simulink model "MOD_Hbridge_Ctrl"  (R2018b)
settings: Solver=VariableStepDiscrete  StartTime=0  StopTime=30  RelTol=1e-3
PreLoadFcn:
  | if(exist('MBDS_ModelCallback', 'file'))
  |    MBDS_ModelCallback('PreLoad');
  | end
PostLoadFcn:
  | if(exist('MBDS_ModelCallback', 'file'))
  |    MBDS_ModelCallback('PostLoad');
  | end
InitFcn:
  | if(exist('MBDS_ModelCallback', 'file'))
  |    MBDS_ModelCallback('Init');
  | end
StartFcn:
  | if(exist('MBDS_ModelCallback', 'file'))
  |    MBDS_ModelCallback('Start');
  | end
StopFcn:
  | if(exist('MBDS_ModelCallback', 'file'))
  |    MBDS_ModelCallback('Stop');
  | end
undefined symbols (not defined in the file): sigbuilder_block
libraries: simulink x1
(part 1 of 2)
PreSaveFcn:
  | if(exist('MBDS_ModelCallback', 'file'))
  |    MBDS_ModelCallback('PreSave');
  | end
CloseFcn:
  | if(exist('MBDS_ModelCallback', 'file'))
  |    MBDS_ModelCallback('Close');
  | end
Description:
  | Design model of an MBDS Module
settings Model: IsTargetCode=false  MBDS_Version=08.20  Creator=Denis Cerchiaro (uidu1522)  LastModifiedBy=uidu1522
settings ConfigSet: Description=MBDS configuration set optimized for simulation of model designs for automotive embedded systems.
settings SolverCC: MinimalZcImpactIntegration=on
settings DataIOCC: MaxDataPoints=100  SaveFormat=StructureWithTime  SaveOutput=off  DSMLogging=off  VisualizeSimOutput=off  SaveTime=off  SignalLoggingName=LogSignals
settings OptimizationCC: UseDivisionForNetSlopeComputation=UseDivisionForReciprocalsOfIntegersOnly  UseFloatMulNetSlope=on  DefaultUnderspecifiedDataType=single  OptimizeBlockIOStorage=off  BufferReuse=off  GlobalBufferReuse=off  StrengthReduction=on  ExpressionFolding=off  ExpressionDepthLimit=2147483647  LocalBlockOutputs=off  EfficientFloat2IntCast=on  LifeSpan=inf  BufferReusableBoundary=off  OptimizeBlockOrder=speed  OptimizeDataStoreBuffers=off  BusAssignmentInplaceUpdate=off  LabelGuidedReuse=on
settings DebuggingCC: SignalInfNanChecking=error  AlgebraicLoopMsg=error  ArtificialAlgebraicLoopMsg=error  UnderspecifiedInitializationDetection=Classic  CheckExecutionContextPreStartOutputMsg=on  CheckExecutionContextRuntimeOutputMsg=on  BlockPriorityViolationMsg=error  MinStepSizeMsg=error  TimeAdjustmentMsg=warning  SolverPrmCheckMsg=error  InheritedTsInSrcMsg=none  SingleTaskRateTransMsg=error  TasksWithSamePriorityMsg=error  SigSpecEnsureSampleTimeMsg=error  CheckMatrixSingularityMsg=error  ParameterUnderflowMsg=error  ParameterTunabilityLossMsg=error  FixptConstUnderflowMsg=warning  FixptConstOverflowMsg=warning  FixptConstPrecisionLossMsg=warning  VectorMatrixConversionMsg=error  SignalLabelMismatchMsg=warning  SFcnCompatibilityMsg=error  FrameProcessingCompatibilityMsg=warning  UniqueDataStoreMsg=error  BusObjectLabelMismatch=error  RootOutportRequireBusObject=error  AllowSymbolicDim=off  ModelReferenceIOMsg=error  ModelReferenceIOMismatchMessage=error  UnknownTsInhSupMsg=error  ModelReferenceDataLoggingMessage=error  StateNameClashWarn=warning  SimStateOlderReleaseMsg=warning  StrictBusMsg=ErrorOnBusTreatedAsVector  NonBusSignalsTreatedAsBus=error  SFInvalidInputDataAccessInChartInitDiag=error  SFTransitionOutsideNaturalParentDiag=error  SFUnreachableExecutionPathDiag=error  SFUndirectedBroadcastEventsDiag=error  SFTransitionActionBeforeConditionDiag=error  SFTemporalDelaySmallerThanSampleTimeDiag=error  SFExecutionAtInitializationDiag=none
settings HardwareCC: ProdBitPerPointer=32  ProdBitPerSizeT=32  ProdBitPerPtrDiffT=32  ProdLargestAtomicInteger=Long  ProdEndianess=BigEndian  ProdWordSize=32  ProdLongLongMode=on  ProdHWDeviceType=Custom Processor  TargetHWDeviceType=32-bit Generic
settings ModelReferenceCC: PropagateSignalLabelsOutOfModel=off
settings SFSimCC: SimUseLocalCustomCode=off  SimGenImportedTypeDefs=on  CompileTimeRecursionLimit=0  EnableRuntimeRecursion=off  MATLABDynamicMemAlloc=off  DefaultCustomCodeFunctionArrayLayout=Column-major
settings RTWCC: SystemTargetFile=MBDS.tlc  GenCodeOnly=on  TemplateMakefile=MBDS.tmf  Description=MBDS Target  GenerateReport=on  RTWUseLocalCustomCode=off  IncludeHyperlinkInReport=on  LaunchReport=on  GenerateTraceReport=on  GenerateTraceReportSl=on  GenerateTraceReportSf=on  GenerateTraceReportEml=on  GenerateCodeMetricsReport=on  RTWCompilerOptimization=on
settings CodeAppCC: ForceParamTrailComments=on  IgnoreCustomStorageClasses=off  OperatorAnnotations=on  SimulinkDataObjDesc=on  SFDataObjDesc=on  MangleLength=2  CustomSymbolStrType=$N$R$M  CustomSymbolStrFcn=$R$M  CustomSymbolStrUtil=$n$C  InsertBlockDesc=on  StateflowObjectComments=on  MATLABSourceComments=on  ReqsInCode=on  UseSimReservedNames=on
settings STFCustomTargetCC: UtilityFuncGeneration=Shared location  MultiwordLength=256  DynamicStringBufferSize=2  InferredTypesCompatibility=on  ModelReferenceCompliant=off  IncludeMdlTerminateFcn=off  CombineOutputUpdateFcns=on  CombineSignalStateStructs=on  SuppressErrorStatus=on  ERTCustomFileBanners=on  SupportComplex=off  SupportContinuousTime=off  SupportNonInlinedSFcns=off  RemoveDisableFunc=on  RemoveResetFunc=on  ParenthesesLevel=Maximum  CastingMode=Standards  MATLABClassNameForMDSCustomization=Simulink.SoftwareTarget.ERTCustomization  GenerateSharedConstants=off  SystemTargetFile=MBDS.tlc
settings ERTTargetCC: UtilityFuncGeneration=Shared location  DynamicStringBufferSize=2  InferredTypesCompatibility=on  ModelReferenceCompliant=off  ParMdlRefBuildCompliant=off  CompOptLevelCompliant=off  ConcurrentExecutionCompliant=off  IncludeMdlTerminateFcn=off  CombineSignalStateStructs=on  SuppressErrorStatus=on  SupportComplex=off  RemoveDisableFunc=on  ParenthesesLevel=Maximum  CastingMode=Standards  ModelStepFunctionPrototypeControlCompliant=off  CPPClassGenCompliant=off  UseToolchainInfoCompliant=off  GenerateSharedConstants=off  ERTCustomFileTemplate=example_file_process.tlc  EnableDataOwnership=on  PreserveExpressionOrder=on  PreserveIfCondition=on  SuppressUnreachableDefaultCases=off  EnableSignedLeftShifts=off  EnableSignedRightShifts=off  IndentStyle=Allman  NewlineStyle=CR+LF
settings ConfigComp: CovScope=ReferencedModels  CovIncludeTopModel=off  CovPath=MOD_Hbridge_Ctrl/Model/MOD_Hbridge_Ctrl_  CovSaveName=covData  CovMetricSettings=dsw  CovFilter=MBDS_CoverageFilter  CovHTMLOptions=-sRT=1 -sVT=0 -aTS=1 -bRG=1 -bTC=1 -hTR=1 -nFC=0 -nFD=0 -scm=1 -bcm=1 -xEv=0 -xEM=1  CovHtmlReporting=on  CovSaveOutputData=off  CovDataFileName=covData  CovShowResultsExplorer=off  CovExternalEMLEnable=off  CovSFcnEnable=off

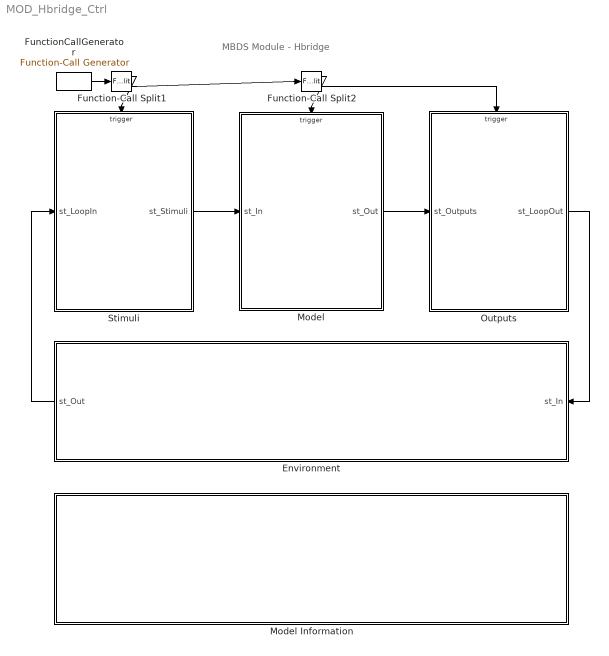
== system MOD_Hbridge_Ctrl ==
  note: MBDS Module - Hbridge
  Environment : Subsystem  Description=Environment subsystem for a MBDS model.
  Function-Call Split1 : FunctionCallSplit  InitFcn=|  NumOutputPorts=2
      | try
      |    MBDS_BlockCallback('Update', gcb);
      | end
      | try
      |    MBDS_BlockCallback('Update', gcb);
      | end
  Function-Call Split2 : FunctionCallSplit  InitFcn=|  NumOutputPorts=2
      | try
      |    MBDS_BlockCallback('Update', gcb);
      | end
      | try
      |    MBDS_BlockCallback('Update', gcb);
      | end
  FunctionCallGenerator : simulink/Ports & Subsystems/Function-Call Generator  sample_time=0.05  numberOfIterations=1
      settings: AttributesFormatString=Ts = %<sample_time>
  Model : Subsystem  Description=Model subsystem for a MBDS model. Here, the input signals to the model functionality are resolved from the Stimuli bus and the output signals of the model functionality are summarized into the Results bus.
  Model Information : Subsystem  InitFcn=|  mask(ModelInformation){MBDS_LibraryBlock=on, Company=-, Department=-, Responsible=-, Status=In Work, Complete=on, Check=on, Test=on, Optimize=on, Documentation=on, FcnErrors=off, GenericToDo=off, DocumentState=Draft, GenericToDoName=Enter a user specific ToDo text, MBDS_BlockVersion=07.00}
      | if(exist('MBDS_BlockCallback', 'file'))
      |    MBDS_BlockCallback('Update', gcb);
      | end
      mask prompts: MBDS_LibraryBlock "MBDS Library Block"; Complete "Complete Implementation"; Check "Check Modelling Guidelines"; Test "Test Functionality"; Optimize "Optimize Implementation"; Documentation "Create Documentation"; FcnErrors "Remove Functional Errors"; GenericToDo "Enter a user specific ToDo text"; DocumentState "Document State:"; GenericToDoName "Generic ToDo Name:"; MBDS_BlockVersion "Block version:"
      mask help: This block displays model information and ToDo's on it's block mask. Via the block parameter mask further model information and configuration options can be accessed.
      mask init:
      | if(exist('MBDS_BlockCallback', 'file'))
      |    MBDS_BlockCallback('Copy', gcb);    
      | end
      mask Help: eval(['open([workdir(''library_dir:''),''\Blockset\help\'',get_param(gcb,''MaskType''),''.html''])'])
      mask TypeOptions Status: In Work | Done
      mask TypeOptions DocumentState: Draft | Final | Released
      mask Callback GenericToDoName:
      | MaskPrompts = get_param(gcb, 'MaskPrompts');
      | MaskPrompts{12} = get_param(gcb, 'GenericToDoName');
      | if(length(MaskPrompts{12}) > 75)
      |    MaskPrompts{12} = MaskPrompts{12}(1:75);
      |    set_param(gcb, 'GenericToDoName', MaskPrompts{12});
      | end
      | set_param(gcb, 'MaskPrompts', MaskPrompts);
      | clear MaskPrompts;
      mask DialogControl ParameterTabVar0 Prompt: Info
      mask DialogControl ParameterTabVar01 Prompt: ToDo's
      mask DialogControl ParameterTabVar012 Prompt: Options
      mask DialogControl ParameterTabVar0123 Prompt: Version
      mask Display:
      | % Get ToDo's
      | IsComplete       = strcmpi(Complete, 'on');
      | IsOptimize       = strcmpi(Optimize, 'on');
      | IsCheck          = strcmpi(Check, 'on');
      | IsDocumentation  = strcmpi(Documentation, 'on');
      | IsTest           = strcmpi(Test, 'on');
      | IsFcnErrors      = strcmpi(FcnErrors, 'on');
      | IsGenericToDo    = strcmpi(GenericToDo, 'on');
      | 
      | % Determine status
      | if(IsFcnErrors || IsTest || IsComplete || IsDocumentation || IsCheck || IsOptimize || IsGenericToDo)
      |    Status = 'In Work';
      | else
      |    Status = 'Done';
      | end
      | 
      | % Update status parameter
      | if(~strcmpi(get_param(gcb, 'Status'), Status))
      |    set_param(gcb, 'Status', Status);
      | end
      | 
      | % Determine severity
      | if(IsFcnErrors)
      |    % Severity: Critical
      |    BoxColorFile = 'Box_Red.tif';
      |    IconFile     = 'State_Red.jpg';
      | elseif (IsTest || IsComplete || IsGenericToDo)
      |    % Severity: Major
      |    BoxColorFile = 'Box_Orange.tif';
      |    IconFile     = 'State_Orange.jpg';
      | elseif (IsDocumentation || IsCheck || IsOptimize)
      |    % Severity: Minor
      |    BoxColorFile = 'Box_Grey.tif';
      |    IconFile     = 'State_Grey.jpg';
      | else
      |    % Severity: None
      |    BoxColorFile = 'Box_Green.tif';
      |    IconFile     = 'State_Green.jpg';
      | end
      | 
      | % Display Model Information
      | InfoStr1 = sprintf('%s', get_param(bdroot, 'Name'));
      | InfoStr2 = sprintf('Model Version:  %s', get_param(bdroot, 'ModelVersion'));
      | InfoStr3 = sprintf('Company:  %s', Company);
      | InfoStr4 = sprintf('Department:  %s', Department);
      | InfoStr5 = sprintf('Responsible:  %s', Responsible);
      | InfoStr6 = sprintf('Last Modified by:  %s at %s', get_param(bdroot, 'LastModifiedBy'), get_param(bdroot, 'LastModifiedDate'));
      | %Y is to do!!!!
      | text(0.5, 0.69, sprintf('%s\n%s\n%s\n%s\n%s\n%s\n%s', InfoStr1, InfoStr2, InfoStr3, InfoStr4, InfoStr5, InfoStr6), 'horizontalAlignment', 'center');
      | clear InfoStr1 InfoStr2 InfoStr3 InfoStr4 InfoStr5 InfoStr6;
      | 
      | % Display Status
      | if(exist(BoxColorFile, 'file'))
      |    image(imread(BoxColorFile,'tif'), [0,0,1,0.45]);
      | end
      | if(exist(IconFile, 'file'))
      |    image(imread(IconFile,'jpg'), [0.025,0.09,0.08,0.26]);
      |    image(imread(IconFile,'jpg'), [0.9,0.09,0.08,0.26]);
      | end
      | plot([-0.01 1.01], [0.45 0.45])
      | text(0.5, 0.38, sprintf('Status: %s', upper(Status)), 'horizontalAlignment', 'center');
      | 
      | % Display ToDo's
      | if(IsComplete)
      |    text(0.15, 0.31, '- Complete Implementation');
      | end
      | if(IsOptimize)
      |    text(0.6, 0.31, '- Optimize Implementation');
      | end
      | 
      | if(IsCheck)
      |    text(0.15, 0.23, '- Check Modeling Guidelines');
      | end
      | if(IsDocumentation)
      |    text(0.6, 0.23, '- Create Documentation');
      | end
      | 
      | if(IsTest)
      |    text(0.15, 0.14, '- Test Functionality');
      | end
      | if(IsFcnErrors)
      |    text(0.6, 0.14, '- Remove Functional Errors');
      | end
      | 
      | if(IsGenericToDo)
      |    text(0.15, 0.06, ['- ', GenericToDoName]);
      | end
  Outputs : Subsystem  Description=Result subsystem for a MBDS model. Here, output signals from the model functionality can be displayed using a scope or display. Additionally, the output signals can be postprocessed before they will passed to the feedback loop.
  Stimuli : Subsystem  Description=Stimuli subsystem for a MBDS model. Here, input signals for testing the model functionality can be defined using the signal builder or calculated applying arbitrary basic-blocks. Additionally, feedback signals can be preprocessed at this stage.
  wires:
  Model/1(st_Out) -> Outputs/1(st_Outputs)
  Stimuli/1(st_Stimuli) -> Model/1(st_In)
  Outputs/1(st_LoopOut) -> Environment/1(st_In)
  Environment/1(st_Out) -> Stimuli/1(st_LoopIn)
  FunctionCallGenerator/1 -> Function-Call Split1/1
  Function-Call Split1/1 -> Stimuli/Trigger
  Function-Call Split2/1 -> Model/Trigger
  Function-Call Split2/2 -> Outputs/Trigger
  Function-Call Split1/2 -> Function-Call Split2/1

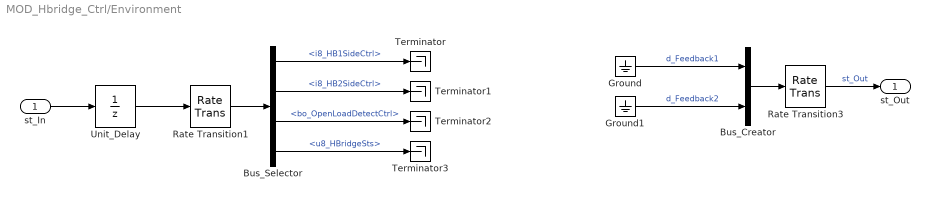
== system MOD_Hbridge_Ctrl/Environment ==
  st_In : Inport
  Bus_Creator : BusCreator  InitFcn=|  Inputs=2
      | try
      |    MBDS_BlockCallback('Update', gcb);
      | end
      | try
      |    MBDS_BlockCallback('Update', gcb);
      | end
  Bus_Selector : BusSelector  InitFcn=|  OutputSignals=i8_HB1SideCtrl,i8_HB2SideCtrl,bo_OpenLoadDetectCtrl,u8_HBridgeSts
      | try
      |    MBDS_BlockCallback('Update', gcb);
      | end
      | try
      |    MBDS_BlockCallback('Update', gcb);
      | end
  Ground : Ground  InitFcn=|
      | try
      |    MBDS_BlockCallback('Update', gcb);
      | end
  Ground1 : Ground  InitFcn=|
      | try
      |    MBDS_BlockCallback('Update', gcb);
      | end
  Rate Transition1 : RateTransition  InitFcn=|  OutPortSampleTimeOpt=Inherit
      | try
      |    MBDS_BlockCallback('Update', gcb);
      | end
  Rate Transition3 : RateTransition  InitFcn=|  OutPortSampleTimeOpt=Inherit
      | try
      |    MBDS_BlockCallback('Update', gcb);
      | end
  Terminator{,1..3} (4 alike) : Terminator
      settings: MoveFcn=UpdateBlockSize(gcb);
      settings: InitFcn=|
      | try
      |    MBDS_BlockCallback('Update', gcb);
      | end
  Unit_Delay : UnitDelay  InitFcn=|  SampleTime=-1
      | try
      |    MBDS_BlockCallback('Update', gcb);
      | end
      | try                                  
      |    MBDS_BlockCallback('Update', gcb);
      | end
      settings: AttributesFormatString=Init = %<X0>
  st_Out : Outport
  wires:
  Bus_Creator/1 -> Rate Transition3/1
  Ground/1 -> Bus_Creator/1  "d_Feedback1"
  Ground1/1 -> Bus_Creator/2  "d_Feedback2"
  Unit_Delay/1 -> Rate Transition1/1
  Rate Transition1/1 -> Bus_Selector/1
  Rate Transition3/1 -> st_Out/1  "st_Out"
  st_In/1 -> Unit_Delay/1
  Bus_Selector/1 -> Terminator/1  "<i8_HB1SideCtrl>"
  Bus_Selector/2 -> Terminator1/1  "<i8_HB2SideCtrl>"
  Bus_Selector/3 -> Terminator2/1  "<bo_OpenLoadDetectCtrl>"
  Bus_Selector/4 -> Terminator3/1  "<u8_HBridgeSts>"

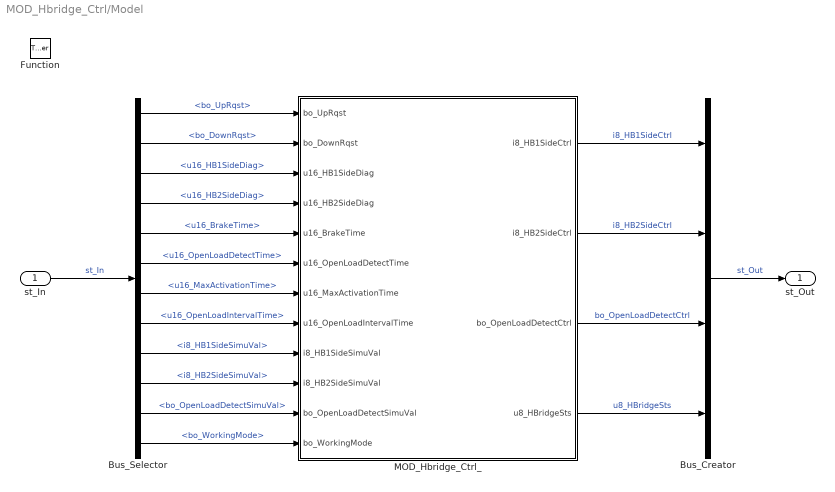
== system MOD_Hbridge_Ctrl/Model ==
  st_In : Inport
      settings: LatchInputForFeedbackSignals=on
  Function : TriggerPort  InitFcn=|  TriggerType=function-call  VariantControl=(inherit)
      | try
      |    MBDS_BlockCallback('Update', gcb);
      | end
  Bus_Creator : BusCreator  InitFcn=|  Inputs=4
      | try
      |    MBDS_BlockCallback('Update', gcb);
      | end
      | try
      |    MBDS_BlockCallback('Update', gcb);
      | end
  Bus_Selector : BusSelector  InitFcn=|  OutputSignals=bo_UpRqst,bo_DownRqst,u16_HB1SideDiag,u16_HB2SideDiag,u16_BrakeTime,u16_OpenLoadDetectTime,u16_MaxActivationTime,u16_OpenLoadIntervalTime,i8_HB1SideSimuVal,i8_HB2SideSimuVal,bo_OpenLoadDetectSimuVal,bo_WorkingMode
      | try
      |    MBDS_BlockCallback('Update', gcb);
      | end
      settings: MoveFcn=UpdateBlockSize(gcb);
  MOD_Hbridge_Ctrl_ : Subsystem  Tag=Functionality  Description=Hbridge
      settings: AttributesFormatString=Functionality
  st_Out : Outport  InitFcn=|
      | try
      |    MBDS_BlockCallback('Update', gcb);
      | end
  wires:
  st_In/1 -> Bus_Selector/1  "st_In"
  Bus_Creator/1 -> st_Out/1  "st_Out"
  Bus_Selector/1 -> MOD_Hbridge_Ctrl_/1(bo_UpRqst)  "<bo_UpRqst>"
  Bus_Selector/2 -> MOD_Hbridge_Ctrl_/2(bo_DownRqst)  "<bo_DownRqst>"
  Bus_Selector/3 -> MOD_Hbridge_Ctrl_/3(u16_HB1SideDiag)  "<u16_HB1SideDiag>"
  Bus_Selector/4 -> MOD_Hbridge_Ctrl_/4(u16_HB2SideDiag)  "<u16_HB2SideDiag>"
  Bus_Selector/5 -> MOD_Hbridge_Ctrl_/5(u16_BrakeTime)  "<u16_BrakeTime>"
  Bus_Selector/6 -> MOD_Hbridge_Ctrl_/6(u16_OpenLoadDetectTime)  "<u16_OpenLoadDetectTime>"
  Bus_Selector/7 -> MOD_Hbridge_Ctrl_/7(u16_MaxActivationTime)  "<u16_MaxActivationTime>"
  Bus_Selector/8 -> MOD_Hbridge_Ctrl_/8(u16_OpenLoadIntervalTime)  "<u16_OpenLoadIntervalTime>"
  Bus_Selector/9 -> MOD_Hbridge_Ctrl_/9(i8_HB1SideSimuVal)  "<i8_HB1SideSimuVal>"
  Bus_Selector/10 -> MOD_Hbridge_Ctrl_/10(i8_HB2SideSimuVal)  "<i8_HB2SideSimuVal>"
  Bus_Selector/11 -> MOD_Hbridge_Ctrl_/11(bo_OpenLoadDetectSimuVal)  "<bo_OpenLoadDetectSimuVal>"
  Bus_Selector/12 -> MOD_Hbridge_Ctrl_/12(bo_WorkingMode)  "<bo_WorkingMode>"
  MOD_Hbridge_Ctrl_/1(i8_HB1SideCtrl) -> Bus_Creator/1  "i8_HB1SideCtrl"
  MOD_Hbridge_Ctrl_/2(i8_HB2SideCtrl) -> Bus_Creator/2  "i8_HB2SideCtrl"
  MOD_Hbridge_Ctrl_/3(bo_OpenLoadDetectCtrl) -> Bus_Creator/3  "bo_OpenLoadDetectCtrl"
  MOD_Hbridge_Ctrl_/4(u8_HBridgeSts) -> Bus_Creator/4  "u8_HBridgeSts"

== system MOD_Hbridge_Ctrl/Model Information ==
  note: Double Click the Model Information block to open the block parameter mask

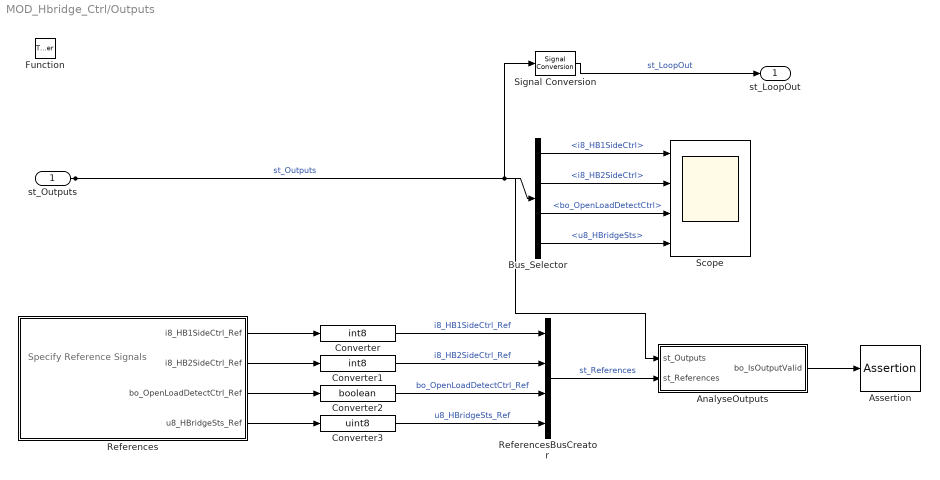
== system MOD_Hbridge_Ctrl/Outputs ==
  note: Specify Reference Signals
  st_Outputs : Inport
      settings: LatchInputForFeedbackSignals=on
  Function : TriggerPort  InitFcn=|  TriggerType=function-call  VariantControl=(inherit)
      | try
      |    MBDS_BlockCallback('Update', gcb);
      | end
  AnalyseOutputs : Subsystem
  Assertion : Assertion  Enabled=off
  Bus_Selector : BusSelector  InitFcn=|  OutputSignals=i8_HB1SideCtrl,i8_HB2SideCtrl,bo_OpenLoadDetectCtrl,u8_HBridgeSts
      | try
      |    MBDS_BlockCallback('Update', gcb);
      | end
      | try
      |    MBDS_BlockCallback('Update', gcb);
      | end
  Converter : DataTypeConversion  InitFcn=|  OutDataTypeStr=int8  SaturateOnIntegerOverflow=on
      | try
      |    MBDS_BlockCallback('Update', gcb);
      | end
      settings: AttributesFormatString=Saturate: %<SaturateOnIntegerOverflow>
  Converter1 : DataTypeConversion  InitFcn=|  OutDataTypeStr=int8  SaturateOnIntegerOverflow=on
      | try
      |    MBDS_BlockCallback('Update', gcb);
      | end
      settings: AttributesFormatString=Saturate: %<SaturateOnIntegerOverflow>
  Converter2 : DataTypeConversion  InitFcn=|  OutDataTypeStr=boolean  SaturateOnIntegerOverflow=on
      | try
      |    MBDS_BlockCallback('Update', gcb);
      | end
      settings: AttributesFormatString=Saturate: %<SaturateOnIntegerOverflow>
  Converter3 : DataTypeConversion  InitFcn=|  OutDataTypeStr=uint8  SaturateOnIntegerOverflow=on
      | try
      |    MBDS_BlockCallback('Update', gcb);
      | end
      settings: AttributesFormatString=Saturate: %<SaturateOnIntegerOverflow>
  References : Subsystem  Tag=STV Subsys  LoadFcn=sigbuilder_block('load');  StartFcn=sigbuilder_block('start');  StopFcn=sigbuilder_block('stop');  ClipboardFcn=sigbuilder_block('clipboard');  mask(Sigbuilder block){tuvar=[0:10]}
      mask init:
      | if ~strcmp(get_param(bdroot(gcb),'SimulationStatus'),'stopped'),tuvar = sigbuilder_block('maskInit'); end
      settings: CopyFcn=sigbuilder_block('copy');  DeleteFcn=sigbuilder_block('delete');  ModelCloseFcn=sigbuilder_block('modelClose');  PreSaveFcn=sigbuilder_block('preSave');  PauseFcn=sigbuilder_block('pause');  ContinueFcn=sigbuilder_block('continue');  NameChangeFcn=sigbuilder_block('namechange');  OpenFcn=sigbuilder_block('open',[50 50 520 400 ]);  CloseFcn=sigbuilder_block('close');
      mask Display: plot(0, 0, 100, 100,[2, 2, 32, 32, 2], [68, 8, 8, 68, 68],[32, 2], [38, 38], [32, 19, 2],[53, 60, 44], [32, 17, 17, 2],[16, 16, 31, 31]);txt = getActiveGroup(gcbh);text(2, 100, txt,'verticalAlignment', 'top');
  ReferencesBusCreator : BusCreator  InitFcn=|  Inputs=4
      | try
      |    MBDS_BlockCallback('Update', gcb);
      | end
      | try
      |    MBDS_BlockCallback('Update', gcb);
      | end
  Scope : Scope  NumInputPorts=4
  Signal Conversion : SignalConversion  InitFcn=|  OverrideOpt=off
      | try
      |    MBDS_BlockCallback('Update', gcb);
      | end
  st_LoopOut : Outport
  wires:
  AnalyseOutputs/1(bo_IsOutputValid) -> Assertion/1
  st_Outputs/1 -> Signal Conversion/1, Bus_Selector/1, AnalyseOutputs/1(st_Outputs)  "st_Outputs"
  Signal Conversion/1 -> st_LoopOut/1  "st_LoopOut"
  Bus_Selector/1 -> Scope/1  "<i8_HB1SideCtrl>"
  Bus_Selector/2 -> Scope/2  "<i8_HB2SideCtrl>"
  Bus_Selector/3 -> Scope/3  "<bo_OpenLoadDetectCtrl>"
  Bus_Selector/4 -> Scope/4  "<u8_HBridgeSts>"
  ReferencesBusCreator/1 -> AnalyseOutputs/2(st_References)  "st_References"
  Converter/1 -> ReferencesBusCreator/1  "i8_HB1SideCtrl_Ref"
  References/1(i8_HB1SideCtrl_Ref) -> Converter/1
  Converter1/1 -> ReferencesBusCreator/2  "i8_HB2SideCtrl_Ref"
  References/2(i8_HB2SideCtrl_Ref) -> Converter1/1
  Converter2/1 -> ReferencesBusCreator/3  "bo_OpenLoadDetectCtrl_Ref"
  References/3(bo_OpenLoadDetectCtrl_Ref) -> Converter2/1
  Converter3/1 -> ReferencesBusCreator/4  "u8_HBridgeSts_Ref"
  References/4(u8_HBridgeSts_Ref) -> Converter3/1

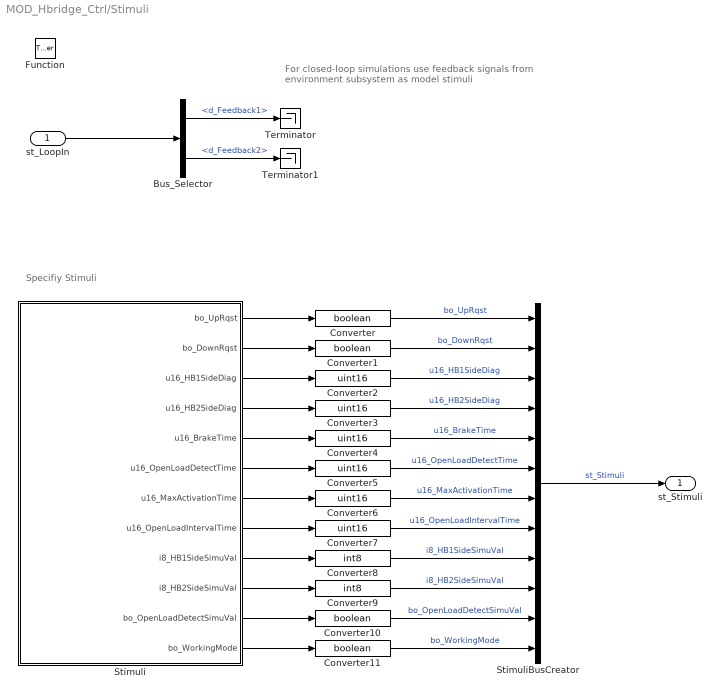
== system MOD_Hbridge_Ctrl/Stimuli ==
  note: Specifiy Stimuli
  note: For closed-loop simulations use feedback signals
      | from environment subsystem as model stimuli
  st_LoopIn : Inport
      settings: LatchInputForFeedbackSignals=on
  Function : TriggerPort  InitFcn=|  TriggerType=function-call  VariantControl=(inherit)
      | try
      |    MBDS_BlockCallback('Update', gcb);
      | end
  Bus_Selector : BusSelector  InitFcn=|  OutputSignals=d_Feedback1,d_Feedback2
      | try
      |    MBDS_BlockCallback('Update', gcb);
      | end
      | try
      |    MBDS_BlockCallback('Update', gcb);
      | end
  Converter : DataTypeConversion  InitFcn=|  OutDataTypeStr=boolean  SaturateOnIntegerOverflow=on
      | try
      |    MBDS_BlockCallback('Update', gcb);
      | end
      settings: AttributesFormatString=Saturate: %<SaturateOnIntegerOverflow>
  Converter1 : DataTypeConversion  InitFcn=|  OutDataTypeStr=boolean  SaturateOnIntegerOverflow=on
      | try
      |    MBDS_BlockCallback('Update', gcb);
      | end
      settings: AttributesFormatString=Saturate: %<SaturateOnIntegerOverflow>
  Converter10 : DataTypeConversion  InitFcn=|  OutDataTypeStr=boolean  SaturateOnIntegerOverflow=on
      | try
      |    MBDS_BlockCallback('Update', gcb);
      | end
      settings: AttributesFormatString=Saturate: %<SaturateOnIntegerOverflow>
  Converter11 : DataTypeConversion  InitFcn=|  OutDataTypeStr=boolean  SaturateOnIntegerOverflow=on
      | try
      |    MBDS_BlockCallback('Update', gcb);
      | end
      settings: AttributesFormatString=Saturate: %<SaturateOnIntegerOverflow>
  Converter2 : DataTypeConversion  InitFcn=|  OutDataTypeStr=uint16  SaturateOnIntegerOverflow=on
      | try
      |    MBDS_BlockCallback('Update', gcb);
      | end
      settings: AttributesFormatString=Saturate: %<SaturateOnIntegerOverflow>
  Converter3 : DataTypeConversion  InitFcn=|  OutDataTypeStr=uint16  SaturateOnIntegerOverflow=on
      | try
      |    MBDS_BlockCallback('Update', gcb);
      | end
      settings: AttributesFormatString=Saturate: %<SaturateOnIntegerOverflow>
  Converter4 : DataTypeConversion  InitFcn=|  OutDataTypeStr=uint16  SaturateOnIntegerOverflow=on
      | try
      |    MBDS_BlockCallback('Update', gcb);
      | end
      settings: AttributesFormatString=Saturate: %<SaturateOnIntegerOverflow>
  Converter5 : DataTypeConversion  InitFcn=|  OutDataTypeStr=uint16  SaturateOnIntegerOverflow=on
      | try
      |    MBDS_BlockCallback('Update', gcb);
      | end
      settings: AttributesFormatString=Saturate: %<SaturateOnIntegerOverflow>
  Converter6 : DataTypeConversion  InitFcn=|  OutDataTypeStr=uint16  SaturateOnIntegerOverflow=on
      | try
      |    MBDS_BlockCallback('Update', gcb);
      | end
      settings: AttributesFormatString=Saturate: %<SaturateOnIntegerOverflow>
  Converter7 : DataTypeConversion  InitFcn=|  OutDataTypeStr=uint16  SaturateOnIntegerOverflow=on
      | try
      |    MBDS_BlockCallback('Update', gcb);
      | end
      settings: AttributesFormatString=Saturate: %<SaturateOnIntegerOverflow>
  Converter8 : DataTypeConversion  InitFcn=|  OutDataTypeStr=int8  SaturateOnIntegerOverflow=on
      | try
      |    MBDS_BlockCallback('Update', gcb);
      | end
      settings: AttributesFormatString=Saturate: %<SaturateOnIntegerOverflow>
  Converter9 : DataTypeConversion  InitFcn=|  OutDataTypeStr=int8  SaturateOnIntegerOverflow=on
      | try
      |    MBDS_BlockCallback('Update', gcb);
      | end
      settings: AttributesFormatString=Saturate: %<SaturateOnIntegerOverflow>
  Stimuli : Subsystem  Tag=STV Subsys  LoadFcn=sigbuilder_block('load');  StartFcn=sigbuilder_block('start');  StopFcn=sigbuilder_block('stop');  ClipboardFcn=sigbuilder_block('clipboard');  mask(Sigbuilder block){tuvar=[0:10]}
      mask init:
      | if ~strcmp(get_param(bdroot(gcb),'SimulationStatus'),'stopped'),tuvar = sigbuilder_block('maskInit'); end
      settings: CopyFcn=sigbuilder_block('copy');  DeleteFcn=sigbuilder_block('delete');  ModelCloseFcn=sigbuilder_block('modelClose');  PreSaveFcn=sigbuilder_block('preSave');  PauseFcn=sigbuilder_block('pause');  ContinueFcn=sigbuilder_block('continue');  NameChangeFcn=sigbuilder_block('namechange');  OpenFcn=sigbuilder_block('open',[6 30 1428 681.75 ]);  CloseFcn=sigbuilder_block('close');
      mask Display: plot(0, 0, 100, 100,[2, 2, 32, 32, 2], [68, 8, 8, 68, 68],[32, 2], [38, 38], [32, 19, 2],[53, 60, 44], [32, 17, 17, 2],[16, 16, 31, 31]);txt = getActiveGroup(gcbh);text(2, 100, txt,'verticalAlignment', 'top');
  StimuliBusCreator : BusCreator  InitFcn=|  Inputs=12
      | try
      |    MBDS_BlockCallback('Update', gcb);
      | end
      | try
      |    MBDS_BlockCallback('Update', gcb);
      | end
  Terminator : Terminator
      settings: InitFcn=|
      | try
      |    MBDS_BlockCallback('Update', gcb);
      | end
      | try
      |    MBDS_BlockCallback('Update', gcb);
      | end
  Terminator1 : Terminator
      settings: InitFcn=|
      | try
      |    MBDS_BlockCallback('Update', gcb);
      | end
      | try
      |    MBDS_BlockCallback('Update', gcb);
      | end
  st_Stimuli : Outport
  wires:
  Bus_Selector/1 -> Terminator/1  "<d_Feedback1>"
  Bus_Selector/2 -> Terminator1/1  "<d_Feedback2>"
  st_LoopIn/1 -> Bus_Selector/1
  StimuliBusCreator/1 -> st_Stimuli/1  "st_Stimuli"
  Converter/1 -> StimuliBusCreator/1  "bo_UpRqst"
  Stimuli/1(bo_UpRqst) -> Converter/1
  Converter1/1 -> StimuliBusCreator/2  "bo_DownRqst"
  Stimuli/2(bo_DownRqst) -> Converter1/1
  Converter2/1 -> StimuliBusCreator/3  "u16_HB1SideDiag"
  Stimuli/3(u16_HB1SideDiag) -> Converter2/1
  Converter3/1 -> StimuliBusCreator/4  "u16_HB2SideDiag"
  Stimuli/4(u16_HB2SideDiag) -> Converter3/1
  Converter4/1 -> StimuliBusCreator/5  "u16_BrakeTime"
  Stimuli/5(u16_BrakeTime) -> Converter4/1
  Converter5/1 -> StimuliBusCreator/6  "u16_OpenLoadDetectTime"
  Stimuli/6(u16_OpenLoadDetectTime) -> Converter5/1
  Converter6/1 -> StimuliBusCreator/7  "u16_MaxActivationTime"
  Stimuli/7(u16_MaxActivationTime) -> Converter6/1
  Converter7/1 -> StimuliBusCreator/8  "u16_OpenLoadIntervalTime"
  Stimuli/8(u16_OpenLoadIntervalTime) -> Converter7/1
  Converter8/1 -> StimuliBusCreator/9  "i8_HB1SideSimuVal"
  Stimuli/9(i8_HB1SideSimuVal) -> Converter8/1
  Converter9/1 -> StimuliBusCreator/10  "i8_HB2SideSimuVal"
  Stimuli/10(i8_HB2SideSimuVal) -> Converter9/1
  Converter10/1 -> StimuliBusCreator/11  "bo_OpenLoadDetectSimuVal"
  Stimuli/11(bo_OpenLoadDetectSimuVal) -> Converter10/1
  Converter11/1 -> StimuliBusCreator/12  "bo_WorkingMode"
  Stimuli/12(bo_WorkingMode) -> Converter11/1

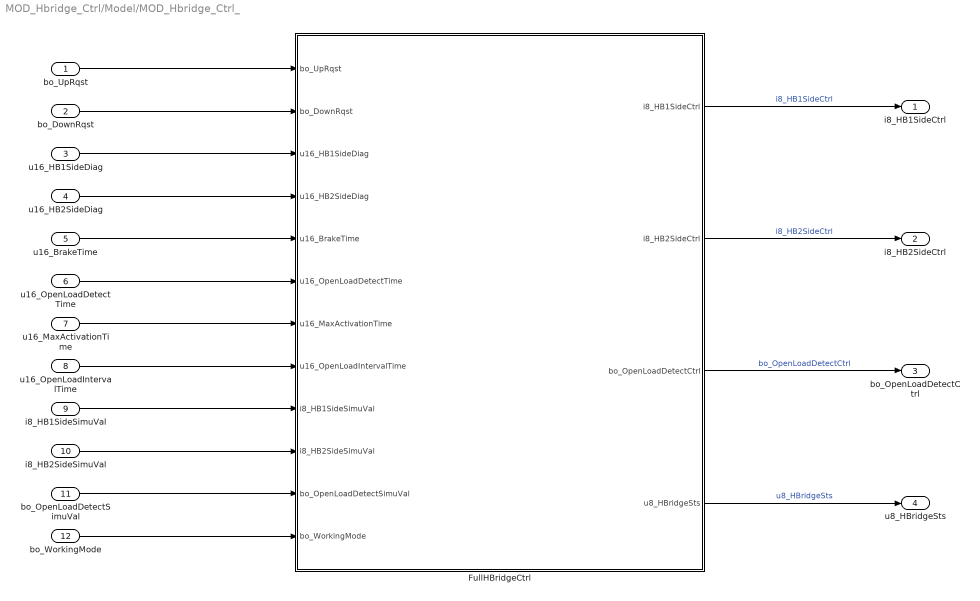
== system MOD_Hbridge_Ctrl/Model/MOD_Hbridge_Ctrl_ ==
  bo_UpRqst : Inport  OutDataTypeStr=boolean
  bo_DownRqst : Inport  Port=2  OutDataTypeStr=boolean
  u16_HB1SideDiag : Inport  Port=3  OutDataTypeStr=uint16
  u16_HB2SideDiag : Inport  Port=4  OutDataTypeStr=uint16
  u16_BrakeTime : Inport  Port=5  OutDataTypeStr=uint16
  u16_OpenLoadDetectTime : Inport  Port=6  OutDataTypeStr=uint16
  u16_MaxActivationTime : Inport  Port=7  OutDataTypeStr=uint16
  u16_OpenLoadIntervalTime : Inport  Port=8  OutDataTypeStr=uint16
  i8_HB1SideSimuVal : Inport  Port=9  OutDataTypeStr=int8
  i8_HB2SideSimuVal : Inport  Port=10  OutDataTypeStr=int8
  bo_OpenLoadDetectSimuVal : Inport  Port=11  OutDataTypeStr=boolean
  bo_WorkingMode : Inport  Port=12  OutDataTypeStr=boolean
  FullHBridgeCtrl : Stateflow chart  TreatAsAtomicUnit=on
      settings: CopyFcn=|
      | if(exist('MBDS_BlockCallback', 'file'))
      |    MBDS_BlockCallback('Copy', gcb);
      | end
  i8_HB1SideCtrl : Outport  OutDataTypeStr=int8
  i8_HB2SideCtrl : Outport  Port=2  OutDataTypeStr=int8
  bo_OpenLoadDetectCtrl : Outport  Port=3  OutDataTypeStr=boolean
  u8_HBridgeSts : Outport  Port=4  OutDataTypeStr=uint8
  wires:
  bo_UpRqst/1 -> FullHBridgeCtrl/1(bo_UpRqst)
  bo_DownRqst/1 -> FullHBridgeCtrl/2(bo_DownRqst)
  u16_HB1SideDiag/1 -> FullHBridgeCtrl/3(u16_HB1SideDiag)
  u16_HB2SideDiag/1 -> FullHBridgeCtrl/4(u16_HB2SideDiag)
  u16_BrakeTime/1 -> FullHBridgeCtrl/5(u16_BrakeTime)
  u16_OpenLoadDetectTime/1 -> FullHBridgeCtrl/6(u16_OpenLoadDetectTime)
  FullHBridgeCtrl/1(i8_HB1SideCtrl) -> i8_HB1SideCtrl/1  "i8_HB1SideCtrl"
  FullHBridgeCtrl/2(i8_HB2SideCtrl) -> i8_HB2SideCtrl/1  "i8_HB2SideCtrl"
  FullHBridgeCtrl/3(bo_OpenLoadDetectCtrl) -> bo_OpenLoadDetectCtrl/1  "bo_OpenLoadDetectCtrl"
  FullHBridgeCtrl/4(u8_HBridgeSts) -> u8_HBridgeSts/1  "u8_HBridgeSts"
  u16_MaxActivationTime/1 -> FullHBridgeCtrl/7(u16_MaxActivationTime)
  u16_OpenLoadIntervalTime/1 -> FullHBridgeCtrl/8(u16_OpenLoadIntervalTime)
  i8_HB1SideSimuVal/1 -> FullHBridgeCtrl/9(i8_HB1SideSimuVal)
  i8_HB2SideSimuVal/1 -> FullHBridgeCtrl/10(i8_HB2SideSimuVal)
  bo_OpenLoadDetectSimuVal/1 -> FullHBridgeCtrl/11(bo_OpenLoadDetectSimuVal)
  bo_WorkingMode/1 -> FullHBridgeCtrl/12(bo_WorkingMode)

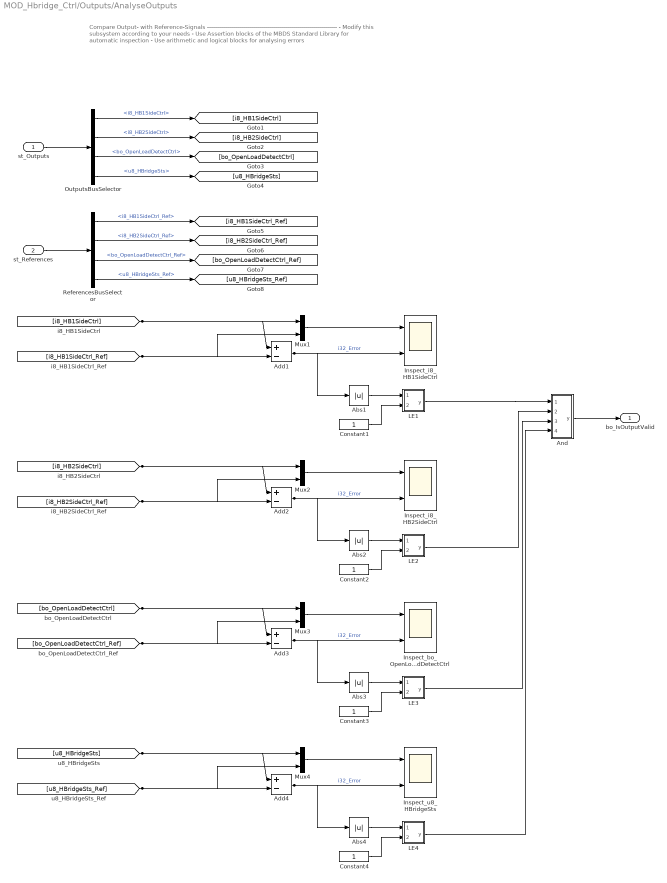
== system MOD_Hbridge_Ctrl/Outputs/AnalyseOutputs ==
  note: Compare Output- with Reference-Signals
      | -----------------------------------------------------------------
      | - Modify this subsystem according to your needs
      | -  Use Assertion blocks of the MBDS Standard Library for automatic inspection
      | - Use arithmetic and logical blocks for analysing errors
  st_Outputs : Inport  InitFcn=|
      | try
      |    MBDS_BlockCallback('Update', gcb);
      | end
  st_References : Inport  InitFcn=|  Port=2
      | try
      |    MBDS_BlockCallback('Update', gcb);
      | end
  Abs1 : Abs  InitFcn=|  OutDataTypeStr=Inherit: Inherit via back propagation
      | if(exist('MBDS_BlockCallback', 'file'))
      |    MBDS_BlockCallback('Update', gcb);  
      | end
      settings: AttributesFormatString=Saturate: %<SaturateOnIntegerOverflow>
  Abs2 : Abs  InitFcn=|  OutDataTypeStr=Inherit: Inherit via back propagation
      | if(exist('MBDS_BlockCallback', 'file'))
      |    MBDS_BlockCallback('Update', gcb);  
      | end
      settings: AttributesFormatString=Saturate: %<SaturateOnIntegerOverflow>
  Abs3 : Abs  InitFcn=|  OutDataTypeStr=Inherit: Inherit via back propagation
      | if(exist('MBDS_BlockCallback', 'file'))
      |    MBDS_BlockCallback('Update', gcb);  
      | end
      settings: AttributesFormatString=Saturate: %<SaturateOnIntegerOverflow>
  Abs4 : Abs  InitFcn=|  OutDataTypeStr=Inherit: Inherit via back propagation
      | if(exist('MBDS_BlockCallback', 'file'))
      |    MBDS_BlockCallback('Update', gcb);  
      | end
      settings: AttributesFormatString=Saturate: %<SaturateOnIntegerOverflow>
  Add1 : Sum  InitFcn=|  Inputs=+-  OutDataTypeStr=int32  SaturateOnIntegerOverflow=on  InputSameDT=on
      | if(exist('MBDS_BlockCallback', 'file'))
      |    MBDS_BlockCallback('Update', gcb);  
      | end
      settings: AttributesFormatString=Saturate: %<SaturateOnIntegerOverflow>
  Add2 : Sum  InitFcn=|  Inputs=+-  OutDataTypeStr=int32  SaturateOnIntegerOverflow=on  InputSameDT=on
      | if(exist('MBDS_BlockCallback', 'file'))
      |    MBDS_BlockCallback('Update', gcb);  
      | end
      settings: AttributesFormatString=Saturate: %<SaturateOnIntegerOverflow>
  Add3 : Sum  InitFcn=|  Inputs=+-  OutDataTypeStr=int32  SaturateOnIntegerOverflow=on  InputSameDT=on
      | if(exist('MBDS_BlockCallback', 'file'))
      |    MBDS_BlockCallback('Update', gcb);  
      | end
      settings: AttributesFormatString=Saturate: %<SaturateOnIntegerOverflow>
  Add4 : Sum  InitFcn=|  Inputs=+-  OutDataTypeStr=int32  SaturateOnIntegerOverflow=on  InputSameDT=on
      | if(exist('MBDS_BlockCallback', 'file'))
      |    MBDS_BlockCallback('Update', gcb);  
      | end
      settings: AttributesFormatString=Saturate: %<SaturateOnIntegerOverflow>
  And : Subsystem  InitFcn=|  mask(AND){MBDS_LibraryBlock=on, BitwiseMode=off, Inputs=4, UseBitMask=off, BitMask='A7', OutDataTypeStr=Inherit: Inherit via back propagation, MBDS_BlockVersion=08.20.02}
      | if(exist('MBDS_BlockCallback', 'file'))
      |    MBDS_BlockCallback('Update', gcb);
      | end
      mask prompts: MBDS_LibraryBlock "MBDS library block"; BitwiseMode "Use 'bitwise' mode"; Inputs "Number of input ports:"; UseBitMask "Use bit mask"; BitMask "Bit mask:"; OutDataTypeStr "Output data type:"; MBDS_BlockVersion "Version:"
      mask help: Logical or bitwise AND operator. For multiple inputs, operators are applied across the inputs. For a single input, operators are applied across the input vector. In bitwise mode a bit mask can be applied onto single input signals.
      mask init:
      | if(exist('MBDS_BlockCallback', 'file'))
      |    MBDS_BlockCallback('Init', gcb);
      | else
      |    % Disable all mask parameters
      |    MaskEnables = get_param(gcb, 'MaskEnables');
      |    for k = [1:length(MaskEnables)]
      |       MaskEnables{k} = 'off';
      |    end
      |    if(~isequal(MaskEnables, get_param(gcb, 'MaskEnables')))
      |       set_param(gcb, 'MaskEnables', MaskEnables);
      |    end
      | end
      mask Help: eval(['open([workdir(''library_dir:''),''\Blockset\help\'',get_param(gcb,''MaskType''),''.html''])'])
      mask Callback BitwiseMode:
      | if(exist('MBDS_BlockCallback', 'file'))
      |    MBDS_BlockCallback('BitwiseMode', gcb);
      | end
      mask Callback Inputs:
      | if(exist('MBDS_BlockCallback', 'file'))
      |    MBDS_BlockCallback('Inputs', gcb);
      | end
      mask Callback UseBitMask:
      | if(exist('MBDS_BlockCallback', 'file'))
      |    MBDS_BlockCallback('UseBitMask', gcb);
      | end
      mask Callback BitMask:
      | if(exist('MBDS_BlockCallback', 'file'))
      |    MBDS_BlockCallback('BitMask', gcb);
      | end
      mask TypeOptions OutDataTypeStr: Inherit: Inherit via back propagation | int8 | uint8 | int16 | uint16 | int32 | uint32 | boolean
      mask Callback OutDataTypeStr:
      | % Adopt Value
      | if(exist('MBDS_BlockCallback', 'file'))
      |    MBDS_BlockCallback('OutDataTypeStr', gcb);
      | end
      mask DialogControl ParameterTabVar0 Prompt: Main
      mask DialogControl ParameterTabVar01 Prompt: Signal Attributes
      mask DialogControl ParameterTabVar012 Prompt: Version
      mask Display:
      | % Show icon or block text
      | if(UseBitMask)
      |    if(isnumeric(BitMask))
      |       BitMaskString = ['0x',dec2hex(floor(BitMask))];
      |    elseif(ischar(BitMask))
      |       BitMaskString = ['0x',upper(BitMask)];
      |    else
      |       BitMaskString = '???';
      |    end
      |    disp(sprintf(['AND\n', BitMaskString]))
      | else
      |    disp('AND')
      | end
  Constant1 : Constant  InitFcn=|  OutDataTypeStr=Inherit: Inherit via back propagation
      | if(exist('MBDS_BlockCallback', 'file'))
      |    MBDS_BlockCallback('Update', gcb);  
      | end
  Constant2 : Constant  InitFcn=|  OutDataTypeStr=Inherit: Inherit via back propagation
      | if(exist('MBDS_BlockCallback', 'file'))
      |    MBDS_BlockCallback('Update', gcb);  
      | end
  Constant3 : Constant  InitFcn=|  OutDataTypeStr=Inherit: Inherit via back propagation
      | if(exist('MBDS_BlockCallback', 'file'))
      |    MBDS_BlockCallback('Update', gcb);  
      | end
  Constant4 : Constant  InitFcn=|  OutDataTypeStr=Inherit: Inherit via back propagation
      | if(exist('MBDS_BlockCallback', 'file'))
      |    MBDS_BlockCallback('Update', gcb);  
      | end
  Inspect_bo_OpenLoadDetectCtrl : Scope  NumInputPorts=2
  Inspect_i8_HB1SideCtrl : Scope  NumInputPorts=2
  Inspect_i8_HB2SideCtrl : Scope  NumInputPorts=2
  Inspect_u8_HBridgeSts : Scope  NumInputPorts=2
  LE1 : Subsystem  InitFcn=|  mask(LE){MBDS_LibraryBlock=on, InputSameDT=on, MBDS_BlockVersion=05.20}
      | if(exist('MBDS_BlockCallback', 'file'))
      |    MBDS_BlockCallback('Update', gcb);
      | end
      mask prompts: MBDS_LibraryBlock "MBDS library block"; InputSameDT "Require all inputs to have the same data type"; MBDS_BlockVersion "Block version:"
      mask help: The block compares if the first input signal is lower than or equal to the second input signal.
      mask init: same as MOD_Hbridge_Ctrl/Outputs/AnalyseOutputs/And
      mask Help: eval(['open([workdir(''library_dir:''),''\Blockset\help\'',get_param(gcb,''MaskType''),''.html''])'])
      mask Callback InputSameDT:
      | % Adopt value
      | if(exist('MBDS_BlockCallback', 'file'))
      |    MBDS_BlockCallback('InputSameDT', gcb);
      | end
      mask DialogControl ParameterTabVar0 Prompt: Signal Attributes
      mask DialogControl ParameterTabVar01 Prompt: Version
      mask Display:
      | % Show icon or block text
      | if(exist('MBDS_BlockCallback', 'file'))
      |    image(imread('LE.tif','tif'),[0.33,0.33,0.37,0.37])
      |    disp('')
      | else
      |    disp(sprintf('<='));
      | end
  LE2 : Subsystem  InitFcn=|  mask(LE){MBDS_LibraryBlock=on, InputSameDT=on, MBDS_BlockVersion=05.20}
      | if(exist('MBDS_BlockCallback', 'file'))
      |    MBDS_BlockCallback('Update', gcb);
      | end
      mask prompts: MBDS_LibraryBlock "MBDS library block"; InputSameDT "Require all inputs to have the same data type"; MBDS_BlockVersion "Block version:"
      mask help: The block compares if the first input signal is lower than or equal to the second input signal.
      mask init: same as MOD_Hbridge_Ctrl/Outputs/AnalyseOutputs/And
      mask Help: eval(['open([workdir(''library_dir:''),''\Blockset\help\'',get_param(gcb,''MaskType''),''.html''])'])
      mask Callback InputSameDT:
      | % Adopt value
      | if(exist('MBDS_BlockCallback', 'file'))
      |    MBDS_BlockCallback('InputSameDT', gcb);
      | end
      mask DialogControl ParameterTabVar0 Prompt: Signal Attributes
      mask DialogControl ParameterTabVar01 Prompt: Version
      mask Display:
      | % Show icon or block text
      | if(exist('MBDS_BlockCallback', 'file'))
      |    image(imread('LE.tif','tif'),[0.33,0.33,0.37,0.37])
      |    disp('')
      | else
      |    disp(sprintf('<='));
      | end
  LE3 : Subsystem  InitFcn=|  mask(LE){MBDS_LibraryBlock=on, InputSameDT=on, MBDS_BlockVersion=05.20}
      | if(exist('MBDS_BlockCallback', 'file'))
      |    MBDS_BlockCallback('Update', gcb);
      | end
      mask prompts: MBDS_LibraryBlock "MBDS library block"; InputSameDT "Require all inputs to have the same data type"; MBDS_BlockVersion "Block version:"
      mask help: The block compares if the first input signal is lower than or equal to the second input signal.
      mask init: same as MOD_Hbridge_Ctrl/Outputs/AnalyseOutputs/And
      mask Help: eval(['open([workdir(''library_dir:''),''\Blockset\help\'',get_param(gcb,''MaskType''),''.html''])'])
      mask Callback InputSameDT:
      | % Adopt value
      | if(exist('MBDS_BlockCallback', 'file'))
      |    MBDS_BlockCallback('InputSameDT', gcb);
      | end
      mask DialogControl ParameterTabVar0 Prompt: Signal Attributes
      mask DialogControl ParameterTabVar01 Prompt: Version
      mask Display:
      | % Show icon or block text
      | if(exist('MBDS_BlockCallback', 'file'))
      |    image(imread('LE.tif','tif'),[0.33,0.33,0.37,0.37])
      |    disp('')
      | else
      |    disp(sprintf('<='));
      | end
  LE4 : Subsystem  InitFcn=|  mask(LE){MBDS_LibraryBlock=on, InputSameDT=on, MBDS_BlockVersion=05.20}
      | if(exist('MBDS_BlockCallback', 'file'))
      |    MBDS_BlockCallback('Update', gcb);
      | end
      mask prompts: MBDS_LibraryBlock "MBDS library block"; InputSameDT "Require all inputs to have the same data type"; MBDS_BlockVersion "Block version:"
      mask help: The block compares if the first input signal is lower than or equal to the second input signal.
      mask init: same as MOD_Hbridge_Ctrl/Outputs/AnalyseOutputs/And
      mask Help: eval(['open([workdir(''library_dir:''),''\Blockset\help\'',get_param(gcb,''MaskType''),''.html''])'])
      mask Callback InputSameDT:
      | % Adopt value
      | if(exist('MBDS_BlockCallback', 'file'))
      |    MBDS_BlockCallback('InputSameDT', gcb);
      | end
      mask DialogControl ParameterTabVar0 Prompt: Signal Attributes
      mask DialogControl ParameterTabVar01 Prompt: Version
      mask Display:
      | % Show icon or block text
      | if(exist('MBDS_BlockCallback', 'file'))
      |    image(imread('LE.tif','tif'),[0.33,0.33,0.37,0.37])
      |    disp('')
      | else
      |    disp(sprintf('<='));
      | end
  Mux1 : Mux  InitFcn=|  Inputs=2
      | try
      |    MBDS_BlockCallback('Update', gcb);
      | end
  Mux2 : Mux  InitFcn=|  Inputs=2
      | try
      |    MBDS_BlockCallback('Update', gcb);
      | end
  Mux3 : Mux  InitFcn=|  Inputs=2
      | try
      |    MBDS_BlockCallback('Update', gcb);
      | end
  Mux4 : Mux  InitFcn=|  Inputs=2
      | try
      |    MBDS_BlockCallback('Update', gcb);
      | end
  OutputsBusSelector : BusSelector  InitFcn=|  OutputSignals=i8_HB1SideCtrl,i8_HB2SideCtrl,bo_OpenLoadDetectCtrl,u8_HBridgeSts
      | try
      |    MBDS_BlockCallback('Update', gcb);
      | end
  ReferencesBusSelector : BusSelector  InitFcn=|  OutputSignals=i8_HB1SideCtrl_Ref,i8_HB2SideCtrl_Ref,bo_OpenLoadDetectCtrl_Ref,u8_HBridgeSts_Ref
      | try
      |    MBDS_BlockCallback('Update', gcb);
      | end
  bo_IsOutputValid : Outport  InitFcn=|  PortDimensions=1
      | try
      |    MBDS_BlockCallback('Update', gcb);
      | end
  wires:
  st_Outputs/1 -> OutputsBusSelector/1
  OutputsBusSelector/1 -> [i8_HB1SideCtrl]  "<i8_HB1SideCtrl>"
  OutputsBusSelector/2 -> [i8_HB2SideCtrl]  "<i8_HB2SideCtrl>"
  OutputsBusSelector/3 -> [bo_OpenLoadDetectCtrl]  "<bo_OpenLoadDetectCtrl>"
  OutputsBusSelector/4 -> [u8_HBridgeSts]  "<u8_HBridgeSts>"
  st_References/1 -> ReferencesBusSelector/1
  ReferencesBusSelector/1 -> [i8_HB1SideCtrl_Ref]  "<i8_HB1SideCtrl_Ref>"
  ReferencesBusSelector/2 -> [i8_HB2SideCtrl_Ref]  "<i8_HB2SideCtrl_Ref>"
  ReferencesBusSelector/3 -> [bo_OpenLoadDetectCtrl_Ref]  "<bo_OpenLoadDetectCtrl_Ref>"
  ReferencesBusSelector/4 -> [u8_HBridgeSts_Ref]  "<u8_HBridgeSts_Ref>"
  [i8_HB1SideCtrl_Ref] -> Add1/2, Mux1/2
  [i8_HB1SideCtrl] -> Add1/1, Mux1/1
  Mux1/1 -> Inspect_i8_HB1SideCtrl/1
  Add1/1 -> Abs1/1, Inspect_i8_HB1SideCtrl/2  "i32_Error"
  Abs1/1 -> LE1/1(u1)
  Constant1/1 -> LE1/2(u2)
  [i8_HB2SideCtrl_Ref] -> Add2/2, Mux2/2
  [i8_HB2SideCtrl] -> Add2/1, Mux2/1
  Mux2/1 -> Inspect_i8_HB2SideCtrl/1
  Add2/1 -> Abs2/1, Inspect_i8_HB2SideCtrl/2  "i32_Error"
  Abs2/1 -> LE2/1(u1)
  Constant2/1 -> LE2/2(u2)
  [bo_OpenLoadDetectCtrl_Ref] -> Add3/2, Mux3/2
  [bo_OpenLoadDetectCtrl] -> Add3/1, Mux3/1
  Mux3/1 -> Inspect_bo_OpenLoadDetectCtrl/1
  Add3/1 -> Abs3/1, Inspect_bo_OpenLoadDetectCtrl/2  "i32_Error"
  Abs3/1 -> LE3/1(u1)
  Constant3/1 -> LE3/2(u2)
  [u8_HBridgeSts_Ref] -> Add4/2, Mux4/2
  [u8_HBridgeSts] -> Add4/1, Mux4/1
  Mux4/1 -> Inspect_u8_HBridgeSts/1
  Add4/1 -> Abs4/1, Inspect_u8_HBridgeSts/2  "i32_Error"
  Abs4/1 -> LE4/1(u1)
  Constant4/1 -> LE4/2(u2)
  And/1(y) -> bo_IsOutputValid/1
  LE1/1(y) -> And/1(u1)
  LE2/1(y) -> And/2(u2)
  LE3/1(y) -> And/3(u3)
  LE4/1(y) -> And/4(u4)

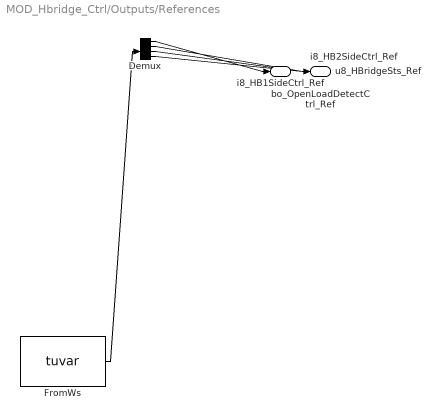
== system MOD_Hbridge_Ctrl/Outputs/References ==
  Demux : Demux  Tag=STV Demux
  FromWs : FromWorkspace  Tag=STV FromWs  VariableName=tuvar
      SigBuilderData=|
      | common.sampleTime = '-1'
      | dataSet(1).timeRange = [0 10]
      | dataSet(1).name = 'TC1'
      | dataSet(2).timeRange = [0 11]
      | dataSet(2).name = 'Test Case 1'
      | dataSet(3).timeRange = [0 10]
      | dataSet(3).name = 'Test Case 2'
      | sbobj.Name = 'Signal Builder'
      | sbobj.Groups(1).Name = 'TC1'
      | sbobj.Groups(1).Signals(1).Name = 'i8_HB1SideCtrl_Ref'
      | sbobj.Groups(1).Signals(1).XData = [0 1 2 3 4 5 6 7 8 9 10]
      | sbobj.Groups(1).Signals(1).YData = [1 1 1 1 1 1 1 1 1 1 1]
      | sbobj.Groups(1).Signals(2).Name = 'i8_HB2SideCtrl_Ref'
      | sbobj.Groups(1).Signals(2).XData = [0 1 2 3 4 5 6 7 8 9 10]
      | sbobj.Groups(1).Signals(2).YData = [1 1 1 1 1 1 1 1 1 1 1]
      | sbobj.Groups(1).Signals(3).Name = 'bo_OpenLoadDetectCtrl_Ref'
      | sbobj.Groups(1).Signals(3).XData = [0 1 2 3 4 4 5 6 6 7 8 9 10]
      | sbobj.Groups(1).Signals(3).YData = [0 0 0 0 0 1 1 1 0 0 0 0 0]
      | sbobj.Groups(1).Signals(4).Name = 'u8_HBridgeSts_Ref'
      | sbobj.Groups(1).Signals(4).XData = [0 1 2 3 4 5 6 7 8 9 10]
      | sbobj.Groups(1).Signals(4).YData = [1 1 1 1 1 1 1 1 1 1 1]
      | sbobj.Groups(2).Name = 'Test Case 1'
      | sbobj.Groups(2).Signals(1).Name = 'i8_HB1SideCtrl_Ref'
      | sbobj.Groups(2).Signals(1).XData = [0 2 2.1 2.1 2.2 2.2 2.3 3 5 5.05 7 7.05 8 8 9 9 10 10 11]
      | sbobj.Groups(2).Signals(1).YData = [0 0 0 1 1 0 0 0 0 0 0 0 0 1 1 -1 -1 1 1]
      | sbobj.Groups(2).Signals(2).Name = 'i8_HB2SideCtrl_Ref'
      | sbobj.Groups(2).Signals(2).XData = [0 2 2.1 2.2 2.2 2.3 2.3 3 5 5 5.05 5.05 7 7 7.05 7.05 8 8 9 9 10 10 11]
      | sbobj.Groups(2).Signals(2).YData = [0 0 0 0 -1 -1 0 0 0 1 1 0 0 1 1 0 0 -1 -1 1 1 -1 -1]
      | sbobj.Groups(2).Signals(3).Name = 'bo_OpenLoadDetectCtrl_Ref'
      | sbobj.Groups(2).Signals(3).XData = [0 2 2 2.1 2.1 2.2 2.3 3 5 5.05 7 7.05 8 9 10 11]
      | sbobj.Groups(2).Signals(3).YData = [0 0 1 1 0 0 0 0 0 0 0 0 0 0 0 0]
      | sbobj.Groups(2).Signals(4).Name = 'u8_HBridgeSts_Ref'
      | sbobj.Groups(2).Signals(4).XData = [0 2 2.1 2.2 2.3 3 5 5.05 7 7.05 8 9 10 11]
      | sbobj.Groups(2).Signals(4).YData = [0 0 0 0 0 0 0 0 0 0 0 0 0 0]
      | sbobj.Groups(2).TimeRange = [0 11]
      | sbobj.Groups(3).Name = 'Test Case 2'
      | sbobj.Groups(3).Signals(1).Name = 'i8_HB1SideCtrl_Ref'
      | sbobj.Groups(3).Signals(1).XData = [0 10]
      | sbobj.Groups(3).Signals(1).YData = [0 0]
      | sbobj.Groups(3).Signals(2).Name = 'i8_HB2SideCtrl_Ref'
      | sbobj.Groups(3).Signals(2).XData = [0 10]
      | sbobj.Groups(3).Signals(2).YData = [0 0]
      | sbobj.Groups(3).Signals(3).Name = 'bo_OpenLoadDetectCtrl_Ref'
      | sbobj.Groups(3).Signals(3).XData = [0 10]
      | sbobj.Groups(3).Signals(3).YData = [0 0]
      | sbobj.Groups(3).Signals(4).Name = 'u8_HBridgeSts_Ref'
      | sbobj.Groups(3).Signals(4).XData = [0 10]
      | sbobj.Groups(3).Signals(4).YData = [0 0]
  i8_HB1SideCtrl_Ref : Outport  Tag=STV Outport
  i8_HB2SideCtrl_Ref : Outport  Tag=STV Outport  Port=2
  bo_OpenLoadDetectCtrl_Ref : Outport  Tag=STV Outport  Port=3
  u8_HBridgeSts_Ref : Outport  Tag=STV Outport  Port=4
  wires:
  FromWs/1 -> Demux/1
  Demux/1 -> i8_HB1SideCtrl_Ref/1
  Demux/2 -> i8_HB2SideCtrl_Ref/1
  Demux/3 -> bo_OpenLoadDetectCtrl_Ref/1
  Demux/4 -> u8_HBridgeSts_Ref/1

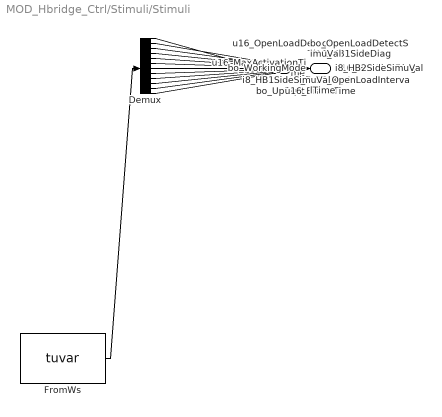
== system MOD_Hbridge_Ctrl/Stimuli/Stimuli ==
  Demux : Demux  Tag=STV Demux  Outputs=12
  FromWs : FromWorkspace  Tag=STV FromWs  VariableName=tuvar
      SigBuilderData=|
      | common.sampleTime = '-1'
      | dataSet(1).timeRange = [0 10]
      | dataSet(1).name = 'TC1'
      | dataSet(2).timeRange = [0 11]
      | dataSet(2).name = 'Test Case 1'
      | dataSet(3).timeRange = [0 10]
      | dataSet(3).name = 'Test Case 2'
      | sbobj.Name = 'Signal Builder'
      | sbobj.Groups(1).Name = 'TC1'
      | sbobj.Groups(1).Signals(1).Name = 'bo_UpRqst'
      | sbobj.Groups(1).Signals(1).XData = [0 1 2 3 4 4 5 6 6 7 8 9 10]
      | sbobj.Groups(1).Signals(1).YData = [0 0 0 0 0 1 1 1 0 0 0 0 0]
      | sbobj.Groups(1).Signals(2).Name = 'bo_DownRqst'
      | sbobj.Groups(1).Signals(2).XData = [0 1 2 3 4 4 5 6 6 7 8 9 10]
      | sbobj.Groups(1).Signals(2).YData = [0 0 0 0 0 1 1 1 0 0 0 0 0]
      | sbobj.Groups(1).Signals(3).Name = 'u16_HB1SideDiag'
      | sbobj.Groups(1).Signals(3).XData = [0 1 2 3 4 5 6 7 8 9 10]
      | sbobj.Groups(1).Signals(3).YData = [1 1 1 1 1 1 1 1 1 1 1]
      | sbobj.Groups(1).Signals(4).Name = 'u16_HB2SideDiag'
      | sbobj.Groups(1).Signals(4).XData = [0 1 2 3 4 5 6 7 8 9 10]
      | sbobj.Groups(1).Signals(4).YData = [1 1 1 1 1 1 1 1 1 1 1]
      | sbobj.Groups(1).Signals(5).Name = 'u16_BrakeTime'
      | sbobj.Groups(1).Signals(5).XData = [0 1 2 3 4 5 6 7 8 9 10]
      | sbobj.Groups(1).Signals(5).YData = [1 1 1 1 1 1 1 1 1 1 1]
      | sbobj.Groups(1).Signals(6).Name = 'u16_OpenLoadDetectTime'
      | sbobj.Groups(1).Signals(6).XData = [0 1 2 3 4 5 6 7 8 9 10]
      | sbobj.Groups(1).Signals(6).YData = [1 1 1 1 1 1 1 1 1 1 1]
      | sbobj.Groups(1).Signals(7).Name = 'u16_MaxActivationTime'
      | sbobj.Groups(1).Signals(7).XData = [0 1 2 3 4 5 6 7 8 9 10]
      | sbobj.Groups(1).Signals(7).YData = [1 1 1 1 1 1 1 1 1 1 1]
      | sbobj.Groups(1).Signals(8).Name = 'u16_OpenLoadIntervalTime'
      | sbobj.Groups(1).Signals(8).XData = [0 1 2 3 4 5 6 7 8 9 10]
      | sbobj.Groups(1).Signals(8).YData = [1 1 1 1 1 1 1 1 1 1 1]
      | sbobj.Groups(1).Signals(9).Name = 'i8_HB1SideSimuVal'
      | sbobj.Groups(1).Signals(9).XData = [0 1 2 3 4 5 6 7 8 9 10]
      | sbobj.Groups(1).Signals(9).YData = [1 1 1 1 1 1 1 1 1 1 1]
      | sbobj.Groups(1).Signals(10).Name = 'i8_HB2SideSimuVal'
      | sbobj.Groups(1).Signals(10).XData = [0 1 2 3 4 5 6 7 8 9 10]
      | sbobj.Groups(1).Signals(10).YData = [1 1 1 1 1 1 1 1 1 1 1]
      | sbobj.Groups(1).Signals(11).Name = 'bo_OpenLoadDetectSimuVal'
      | sbobj.Groups(1).Signals(11).XData = [0 1 2 3 4 4 5 6 6 7 8 9 10]
      | sbobj.Groups(1).Signals(11).YData = [0 0 0 0 0 1 1 1 0 0 0 0 0]
      | sbobj.Groups(1).Signals(12).Name = 'bo_WorkingMode'
      | sbobj.Groups(1).Signals(12).XData = [0 1 2 3 4 4 5 6 6 7 8 9 10]
      | sbobj.Groups(1).Signals(12).YData = [0 0 0 0 0 1 1 1 0 0 0 0 0]
      | sbobj.Groups(2).Name = 'Test Case 1'
      | sbobj.Groups(2).Signals(1).Name = 'bo_UpRqst'
      | sbobj.Groups(2).Signals(1).XData = [0 2 2.1 2.2 2.3 3 5 5.05 7 7.05 8 8 9 9 10 10 11]
      | sbobj.Groups(2).Signals(1).YData = [0 0 0 0 0 0 0 0 0 0 0 1 1 0 0 1 1]
      | sbobj.Groups(2).Signals(2).Name = 'bo_DownRqst'
      | sbobj.Groups(2).Signals(2).XData = [0 2 2.1 2.2 2.3 3 5 5.05 7 7.05 8 9 9 10 10 11]
      | sbobj.Groups(2).Signals(2).YData = [0 0 0 0 0 0 0 0 0 0 0 0 1 1 0 0]
      | sbobj.Groups(2).Signals(3).Name = 'u16_HB1SideDiag'
      | sbobj.Groups(2).Signals(3).XData = [0 2 2.1 2.2 2.3 3 5 5.05 7 7.05 8 9 10 11]
      | sbobj.Groups(2).Signals(3).YData = [0 0 0 0 0 0 0 0 0 0 0 0 0 0]
      | sbobj.Groups(2).Signals(4).Name = 'u16_HB2SideDiag'
      | sbobj.Groups(2).Signals(4).XData = [0 2 2.1 2.2 2.3 3 5 5.05 7 7.05 8 9 10 11]
      | sbobj.Groups(2).Signals(4).YData = [0 0 0 0 0 0 0 0 0 0 0 0 0 0]
      | sbobj.Groups(2).Signals(5).Name = 'u16_BrakeTime'
      | sbobj.Groups(2).Signals(5).XData = [0 2 2.1 2.2 2.3 3 5 5.05 7 7.05 8 9 10 11]
      | sbobj.Groups(2).Signals(5).YData = [10 10 10 10 10 10 10 10 10 10 10 10 10 10]
      | sbobj.Groups(2).Signals(6).Name = 'u16_OpenLoadDetectTime'
      | sbobj.Groups(2).Signals(6).XData = [0 2 2.1 2.2 2.3 3 5 5.05 7 7.05 8 9 10 11]
      | sbobj.Groups(2).Signals(6).YData = [2 2 2 2 2 2 2 2 2 2 2 2 2 2]
      | sbobj.Groups(2).Signals(7).Name = 'u16_MaxActivationTime'
      | sbobj.Groups(2).Signals(7).XData = [0 2 2.1 2.2 2.3 3 5 5.05 7 7.05 8 9 10 11]
      | sbobj.Groups(2).Signals(7).YData = [200 200 200 200 200 200 200 200 200 200 200 200 200 200]
      | sbobj.Groups(2).Signals(8).Name = 'u16_OpenLoadIntervalTime'
      | sbobj.Groups(2).Signals(8).XData = [0 2 2.1 2.2 2.3 3 5 5.05 7 7.05 8 9 10 11]
      | sbobj.Groups(2).Signals(8).YData = [40 40 40 40 40 40 40 40 40 40 40 40 40 40]
      | sbobj.Groups(2).Signals(9).Name = 'i8_HB1SideSimuVal'
      | sbobj.Groups(2).Signals(9).XData = [0 2 2.1 2.1 2.2 2.2 2.3 3 5 5.05 7 7.05 8 9 10 11]
      | sbobj.Groups(2).Signals(9).YData = [0 0 0 1 1 0 0 0 0 0 0 0 0 0 0 0]
      | sbobj.Groups(2).Signals(10).Name = 'i8_HB2SideSimuVal'
      | sbobj.Groups(2).Signals(10).XData = [0 2 2.1 2.2 2.2 2.3 2.3 3 5 5.05 7 7.05 8 9 10 11]
      | sbobj.Groups(2).Signals(10).YData = [0 0 0 0 -1 -1 0 0 0 0 0 0 0 0 0 0]
      | sbobj.Groups(2).Signals(11).Name = 'bo_OpenLoadDetectSimuVal'
      | sbobj.Groups(2).Signals(11).XData = [0 2 2 2.1 2.1 2.2 2.3 3 5 5.05 7 7.05 8 9 10 11]
      | sbobj.Groups(2).Signals(11).YData = [0 0 1 1 0 0 0 0 0 0 0 0 0 0 0 0]
      | sbobj.Groups(2).Signals(12).Name = 'bo_WorkingMode'
      | sbobj.Groups(2).Signals(12).XData = [0 2 2.1 2.2 2.3 3 3 5 5.05 7 7.05 8 9 10 11]
      | sbobj.Groups(2).Signals(12).YData = [0 0 0 0 0 0 1 1 1 1 1 1 1 1 1]
      | sbobj.Groups(2).TimeRange = [0 11]
      | sbobj.Groups(3).Name = 'Test Case 2'
      | sbobj.Groups(3).Signals(1).Name = 'bo_UpRqst'
      | sbobj.Groups(3).Signals(1).XData = [0 10]
      | sbobj.Groups(3).Signals(1).YData = [0 0]
      | sbobj.Groups(3).Signals(2).Name = 'bo_DownRqst'
      | sbobj.Groups(3).Signals(2).XData = [0 10]
      | sbobj.Groups(3).Signals(2).YData = [0 0]
      | sbobj.Groups(3).Signals(3).Name = 'u16_HB1SideDiag'
      | sbobj.Groups(3).Signals(3).XData = [0 10]
      | sbobj.Groups(3).Signals(3).YData = [0 0]
      | sbobj.Groups(3).Signals(4).Name = 'u16_HB2SideDiag'
      | sbobj.Groups(3).Signals(4).XData = [0 10]
      | sbobj.Groups(3).Signals(4).YData = [0 0]
      | sbobj.Groups(3).Signals(5).Name = 'u16_BrakeTime'
      | sbobj.Groups(3).Signals(5).XData = [0 10]
      | sbobj.Groups(3).Signals(5).YData = [0 0]
      | sbobj.Groups(3).Signals(6).Name = 'u16_OpenLoadDetectTime'
      | sbobj.Groups(3).Signals(6).XData = [0 10]
      | sbobj.Groups(3).Signals(6).YData = [0 0]
      | sbobj.Groups(3).Signals(7).Name = 'u16_MaxActivationTime'
      | sbobj.Groups(3).Signals(7).XData = [0 10]
      | sbobj.Groups(3).Signals(7).YData = [0 0]
      | sbobj.Groups(3).Signals(8).Name = 'u16_OpenLoadIntervalTime'
      | sbobj.Groups(3).Signals(8).XData = [0 10]
      | sbobj.Groups(3).Signals(8).YData = [0 0]
      | sbobj.Groups(3).Signals(9).Name = 'i8_HB1SideSimuVal'
      | sbobj.Groups(3).Signals(9).XData = [0 10]
      | sbobj.Groups(3).Signals(9).YData = [0 0]
      | sbobj.Groups(3).Signals(10).Name = 'i8_HB2SideSimuVal'
      | sbobj.Groups(3).Signals(10).XData = [0 10]
      | sbobj.Groups(3).Signals(10).YData = [0 0]
      | sbobj.Groups(3).Signals(11).Name = 'bo_OpenLoadDetectSimuVal'
      | sbobj.Groups(3).Signals(11).XData = [0 10]
      | sbobj.Groups(3).Signals(11).YData = [0 0]
      | sbobj.Groups(3).Signals(12).Name = 'bo_WorkingMode'
      | sbobj.Groups(3).Signals(12).XData = [0 10]
      | sbobj.Groups(3).Signals(12).YData = [0 0]
  bo_UpRqst : Outport  Tag=STV Outport
  bo_DownRqst : Outport  Tag=STV Outport  Port=2
  u16_HB1SideDiag : Outport  Tag=STV Outport  Port=3
  u16_HB2SideDiag : Outport  Tag=STV Outport  Port=4
  u16_BrakeTime : Outport  Tag=STV Outport  Port=5
  u16_OpenLoadDetectTime : Outport  Tag=STV Outport  Port=6
  u16_MaxActivationTime : Outport  Tag=STV Outport  Port=7
  u16_OpenLoadIntervalTime : Outport  Tag=STV Outport  Port=8
  i8_HB1SideSimuVal : Outport  Tag=STV Outport  Port=9
  i8_HB2SideSimuVal : Outport  Tag=STV Outport  Port=10
  bo_OpenLoadDetectSimuVal : Outport  Tag=STV Outport  Port=11
  bo_WorkingMode : Outport  Tag=STV Outport  Port=12
  wires:
  FromWs/1 -> Demux/1
  Demux/1 -> bo_UpRqst/1
  Demux/2 -> bo_DownRqst/1
  Demux/3 -> u16_HB1SideDiag/1
  Demux/4 -> u16_HB2SideDiag/1
  Demux/5 -> u16_BrakeTime/1
  Demux/6 -> u16_OpenLoadDetectTime/1
  Demux/7 -> u16_MaxActivationTime/1
  Demux/8 -> u16_OpenLoadIntervalTime/1
  Demux/9 -> i8_HB1SideSimuVal/1
  Demux/10 -> i8_HB2SideSimuVal/1
  Demux/11 -> bo_OpenLoadDetectSimuVal/1
  Demux/12 -> bo_WorkingMode/1

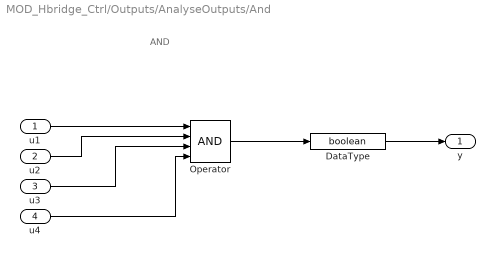
== system MOD_Hbridge_Ctrl/Outputs/AnalyseOutputs/And ==
  note: AND
  u1 : Inport  OutDataTypeStr=boolean
  u2 : Inport  Port=2  OutDataTypeStr=boolean
  u3 : Inport  Port=3  OutDataTypeStr=boolean
  u4 : Inport  Port=4  OutDataTypeStr=boolean
  DataType : DataTypeConversion  OutDataTypeStr=boolean
  Operator : Logic  Inputs=4  AllPortsSameDT=off  OutDataTypeStr=boolean
  y : Outport
  wires:
  Operator/1 -> DataType/1
  u1/1 -> Operator/1
  u2/1 -> Operator/2
  DataType/1 -> y/1
  u3/1 -> Operator/3
  u4/1 -> Operator/4

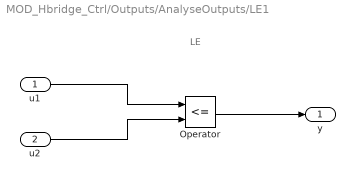
== system MOD_Hbridge_Ctrl/Outputs/AnalyseOutputs/LE1 ==
  note: LE
  u1 : Inport
  u2 : Inport  Port=2
  Operator : RelationalOperator  Operator=<=  OutDataTypeStr=boolean  RndMeth=Nearest  InputSameDT=on
  y : Outport
  wires:
  Operator/1 -> y/1
  u2/1 -> Operator/2
  u1/1 -> Operator/1

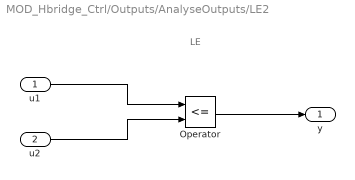
== system MOD_Hbridge_Ctrl/Outputs/AnalyseOutputs/LE2 ==
  note: LE
  u1 : Inport
  u2 : Inport  Port=2
  Operator : RelationalOperator  Operator=<=  OutDataTypeStr=boolean  RndMeth=Nearest  InputSameDT=on
  y : Outport
  wires:
  Operator/1 -> y/1
  u2/1 -> Operator/2
  u1/1 -> Operator/1

== system MOD_Hbridge_Ctrl/Outputs/AnalyseOutputs/LE3 ==
  note: LE
  u1 : Inport
  u2 : Inport  Port=2
  Operator : RelationalOperator  Operator=<=  OutDataTypeStr=boolean  RndMeth=Nearest  InputSameDT=on
  y : Outport
  wires:
  Operator/1 -> y/1
  u2/1 -> Operator/2
  u1/1 -> Operator/1

== system MOD_Hbridge_Ctrl/Outputs/AnalyseOutputs/LE4 ==
  note: LE
  u1 : Inport
  u2 : Inport  Port=2
  Operator : RelationalOperator  Operator=<=  OutDataTypeStr=boolean  RndMeth=Nearest  InputSameDT=on
  y : Outport
  wires:
  Operator/1 -> y/1
  u2/1 -> Operator/2
  u1/1 -> Operator/1
